simulink model "det3x3_HDL"  (R2024a)
settings: Solver=VariableStepAuto  StartTime=0.0  StopTime=100e-9  RelTol=1e-3
undefined symbols (not defined in the file or in its folder): S, vsva2197, xcvc1902
libraries: hdlBasic x32, hdlSSR x1, vmcUtilities x1
settings Model: Creator=catalinb  LastModifiedBy=sdegala
settings DebuggingCC: UnconnectedInputMsg=warning  UnconnectedOutputMsg=warning  UnconnectedLineMsg=warning
settings ModelReferenceCC: EnableRefExpFcnMdlSchedulingChecks=on
settings RTWCC: GPUComputeCapability=3.5  DLArmComputeVersion=19.05

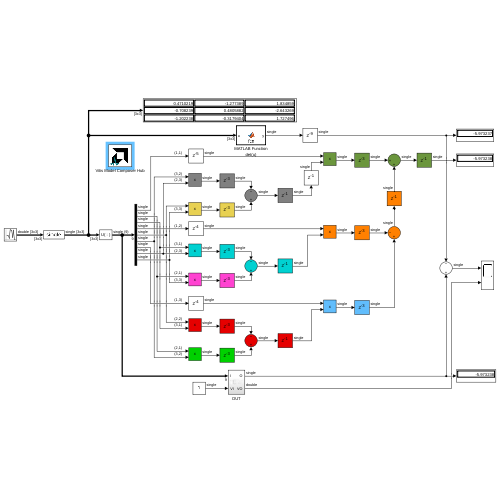
[thumbnail: Simulink's stored preview of the top-level diagram]
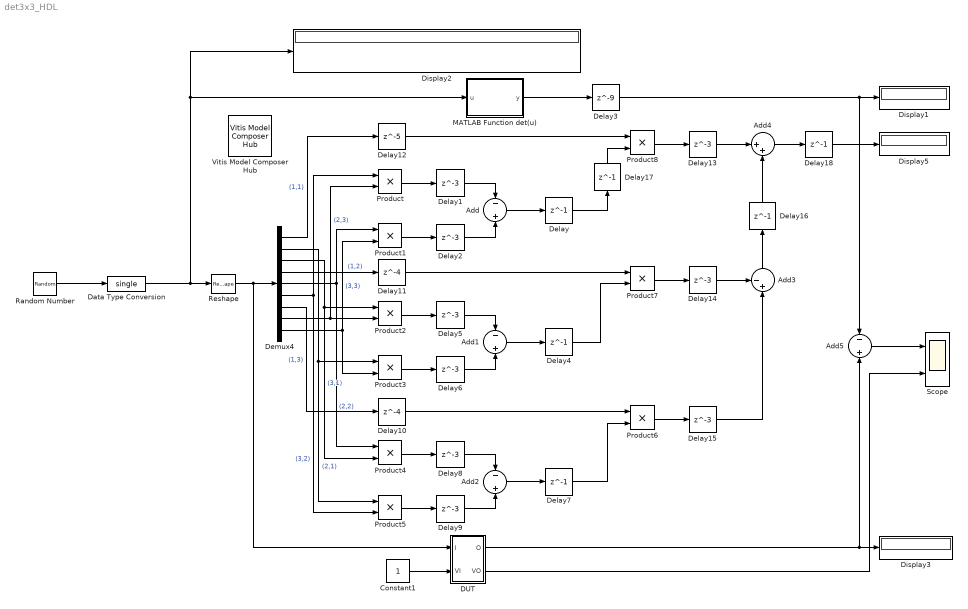
== system det3x3_HDL ==
  Add{,1..2,5} (4 alike) : Sum  Inputs=-|+
  Add3 : Sum  Inputs=-+|
  Add4 : Sum  Inputs=|++
  Constant1 : Constant  OutDataTypeStr=single  SampleTime=1/805e6
  DUT : Subsystem
  Data Type Conversion : DataTypeConversion  OutDataTypeStr=single  SaturateOnIntegerOverflow=off  RndMeth=Floor
  Delay{,4,7,16..18} (6 alike) : Delay  DelayLength=1
  Delay{1..2,5..6,8..9,13..15} (9 alike) : Delay  DelayLength=3
  Delay10 : Delay  DelayLength=4
  Delay11 : Delay  DelayLength=4
  Delay12 : Delay  DelayLength=5
  Delay3 : Delay  DelayLength=9
  Demux4 : Demux  Outputs=9
  Display{1..3,5} (4 alike) : Display
  MATLAB Function det(u) : MATLAB Function  TreatAsAtomicUnit=on
  Product{,1..8} (9 alike) : Product
  Random Number : RandomNumber  Mean=zeros(3,3)  Variance=ones(3,3)  Seed=reshape(1:9,3,3)  SampleTime=1.242e-9  VectorParams1D=off
  Reshape : Reshape
  Scope : Scope  NumInputPorts=2
  Vitis Model Composer Hub : vmcUtilities/Vitis Model Composer Hub  Tag=genX  CodeGeneration=off  SubsystemName=DUT  BlockHierPath=det3x3_HDL/DUT  CompilationType=HDLCompilation  SubsystemType=HDLNode  ExportTypeV2=IP Catalog  StartColumn=1  NumberOfColumns=1  TargetDirectory=./netlist  exportDesign=on  analyzeDesign=off  validateDesignOnHw=off  ExportType=HDL  IpVendor=xilinx.com  IpLibrary=hls  IpVersion=1.0  IpHWLanguage=Verilog  AieCompilerOptions={}  AieSimulatorOptions={}  CreateTestbench=on  TestbenchStackSize=10  RunRtlSim=off  RunCSim=off  RunAieSim=off  AieSimTimeout=50000  RunAieSimProfiling=off  LaunchVitisAnalyzer=off  PlotOutput=off  RunX86Sim=off  X86SimTimeout=10  GenHwImage=off  GenLibadfXo=on  GenHwValidationCode=off  PlatformType=Specify Platform  Platform=/proj/xbuilds/SWIP/9999.0_0905_1841/installs/lin64/2025.2/Vitis/base_platforms/xilinx_vck190_base_202520_1/xilinx_vck190_base_202520_1.xpfm  HwSystemType=Baremetal  HwValidationTarget=hw  ProjDevice=Versal VCK190 Evaluation Platform (xcvc1902-vsva2197-2MP-e-S)  ProjDevicePart=xcvc1902-vsva2197-2MP-e-S  AIEType=AIE  SamplePeriod=-1  ClockFrequency=200  DataPathParallelism=1  xilinxfamily=versalaicore  part=xcvc1902  speed=-2MP-e-S  package=vsva2197  directory=./netlist/ip/DUT/src  testbench=on  incr_netlist=off  synthesis_tool=Vivado  clock_wrapper=Clock Enables  dbl_ovrd=According to Block Masks  dcm_input_clock_period=10  sysclk_period=1.242  simulink_period=1.242e-9  eval_field=0  IPInfoJsonString="{\"DUTSubsystemName\":\"DUT\",\"HDLSubsystem\":{\"SubsystemName\":\"DUT\",\"IPName\":\"Subsystem\",\"IPLibrary\":\"VMC\",\"IPVendor\":\"User Company\",\"IPVersion\":\"1.0\",\"TargetDirectory\":\"./netlist\",\"SubsystemDir\":\"./netlist/ip/DUT\",\"FreqHz\":\"805152979.066\"},\"SubsystemTag\":\"HDLNode\"}"  LogFileName=/proj/xhdhdstaff5/sdegala/Head1/HEAD/ModelComposer_Sept16/Vitis_Model_Composer/Examples/HDL/Floating_Point/3x3_Matrix_Determinant/netlist/model_composer.log  NThreads=4  IPConfigFile=/tmp/vmctmp-9769773316677438567/det3x3_HDL_ipconfig.json
  wires:
  Add/1 -> Delay/1
  Product/1 -> Delay1/1
  Delay1/1 -> Add/1
  Product1/1 -> Delay2/1
  Delay2/1 -> Add/2
  Delay/1 -> Delay17/1
  MATLAB Function det(u)/1(y) -> Delay3/1
  Delay3/1 -> Add5/1, Display1/1
  Reshape/1 -> DUT/1(" I "), Demux4/1
  Demux4/1 -> Delay12/1  "(1,1)"
  Demux4/4 -> Delay11/1  "(1,2)"
  Demux4/7 -> Delay10/1  "(1,3)"
  Demux4/2 -> Product3/1, Product5/1  "(2,1)"
  Demux4/5 -> Product4/1, Product1/1  "(2,2)"
  Demux4/9 -> Product3/2, Product1/2  "(3,3)"
  Demux4/6 -> Product/1, Product5/2  "(3,2)"
  Demux4/8 -> Product/2, Product2/2  "(2,3)"
  Random Number/1 -> Data Type Conversion/1
  Delay4/1 -> Product7/2
  Delay6/1 -> Add1/2
  Product3/1 -> Delay6/1
  Delay5/1 -> Add1/1
  Product2/1 -> Delay5/1
  Add1/1 -> Delay4/1
  Demux4/3 -> Product4/2, Product2/1  "(3,1)"
  Add2/1 -> Delay7/1
  Product4/1 -> Delay8/1
  Delay8/1 -> Add2/1
  Product5/1 -> Delay9/1
  Delay9/1 -> Add2/2
  Delay7/1 -> Product6/2
  Delay10/1 -> Product6/1
  Delay11/1 -> Product7/1
  Delay12/1 -> Product8/1
  Product8/1 -> Delay13/1
  Product7/1 -> Delay14/1
  Product6/1 -> Delay15/1
  Delay14/1 -> Add3/1
  Delay15/1 -> Add3/2
  Add4/1 -> Delay18/1
  Delay16/1 -> Add4/2
  Add3/1 -> Delay16/1
  Delay13/1 -> Add4/1
  Delay18/1 -> Display5/1
  Delay17/1 -> Product8/2
  Constant1/1 -> DUT/2(" VI ")
  DUT/1(" O ") -> Add5/2, Display3/1
  Add5/1 -> Scope/1
  Data Type Conversion/1 -> MATLAB Function det(u)/1(u), Display2/1, Reshape/1
  DUT/2(" VO ") -> Scope/2

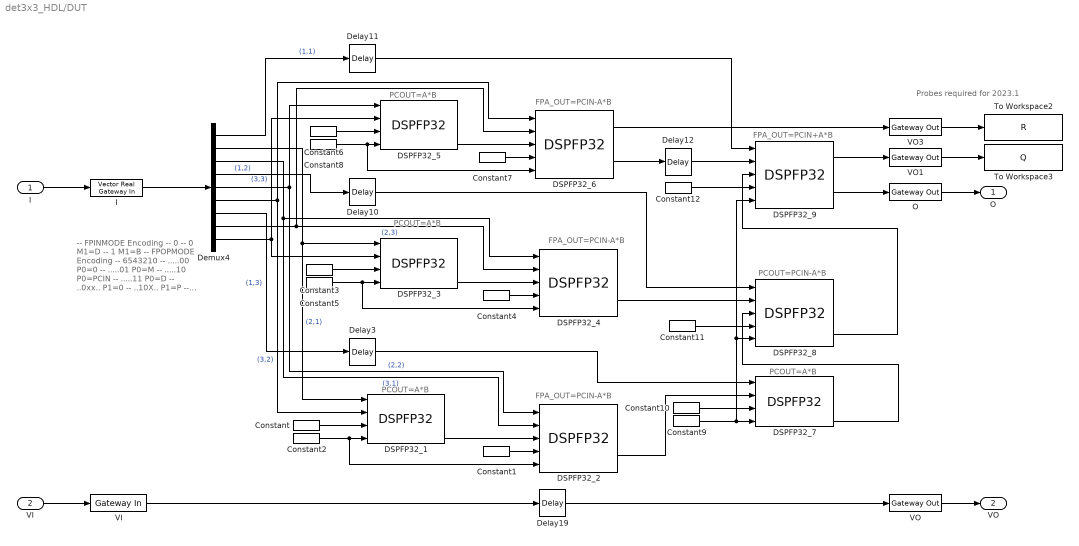
== system det3x3_HDL/DUT ==
  note: Probes required for 2023.1
  note: FPA_OUT=PCIN-A*B
  note: PCOUT=A*B
  note: -- FPINMODE Encoding
      | -- 0
      | -- 0 M1=D
      | -- 1 M1=B
      |
      | -- FPOPMODE Encoding
      | -- 6543210
      | -- .....00 P0=0
      | -- .....01 P0=M
      | -- .....10 P0=PCIN
      | -- .....11 P0=D
      |
      | -- ..0xx.. P1=0
      | -- ..10X.. P1=P
      | -- ..110.. P1=C
      | -- ..111.. P1=PCIN
      |
      | -- 00..... FPA_OUT=P0+P1
      | -- 01..... FPA_OUT=-P0+P1
      | -- 10..... FPA_OUT=P0-P1
      | -- 11..... FPA_OUT=-P0-P1
  note: PCOUT=A*B
  note: PCOUT=PCIN-A*B
  note: FPA_OUT=PCIN+A*B
  note: PCOUT=A*B
  note: PCOUT=A*B
  note: FPA_OUT=PCIN-A*B
  note: FPA_OUT=PCIN-A*B
  " I " : Inport
  " VI " : Inport  Port=2
  Constant{,3,6,10} (4 alike) : hdlBasic/Constant  const=1  gui_display_data_type=Fixed-point  arith_type=Unsigned  n_bits=7  bin_pt=0  preci_type=Single  exp_width=8  frac_width=24  explicit_period=off  period=1  XmcBlockStatus=1  maskContainerNames=tabcontainer1  block_type=constant  block_config=sysgen:Constant_config
  Constant{1,4,7,11} (4 alike) : hdlBasic/Constant  const=61  gui_display_data_type=Fixed-point  arith_type=Unsigned  n_bits=7  bin_pt=0  preci_type=Single  exp_width=8  frac_width=24  explicit_period=off  period=1  XmcBlockStatus=1  maskContainerNames=tabcontainer1  block_type=constant  block_config=sysgen:Constant_config
  Constant12 : hdlBasic/Constant  const=29  gui_display_data_type=Fixed-point  arith_type=Unsigned  n_bits=7  bin_pt=0  preci_type=Single  exp_width=8  frac_width=24  explicit_period=off  period=1  XmcBlockStatus=1  maskContainerNames=tabcontainer1  block_type=constant  block_config=sysgen:Constant_config
  Constant{2,5,8..9} (4 alike) : hdlBasic/Constant  const=1  gui_display_data_type=Fixed-point  arith_type=Unsigned  n_bits=1  bin_pt=0  preci_type=Single  exp_width=8  frac_width=24  explicit_period=off  period=1  XmcBlockStatus=1  maskContainerNames=tabcontainer1  block_type=constant  block_config=sysgen:Constant_config
  DSPFP32_{1,3,5,7} (4 alike) : hdlBasic/DSPFP32   use_a=Direct from a port  use_b=Direct from b port  a_fptype=B32  b_d_fptype=B32  xl_useadderonly=off  xl_dynamicmult=off  use_c=off  use_d=off  rst_all=off  en_all=off  use_pcin=off  use_fpainvalid=off  use_fpaoverflow=off  use_fpaunderflow=off  use_fpminvalid=off  use_fpmoverflow=off  use_fpmunderflow=off  use_acout=off  use_bcout=off  bcascsel=B  use_pcout=on  pcoutsel=FPM  pipeline_a=1  pipeline_acout=1  pipeline_fpcreg=3  pipeline_fpopmreg=1  pipeline_fpbreg=on  pipeline_fpa_preg=on  pipeline_fpm_preg=on  pipeline_fpdreg=on  pipeline_fpmpipereg=on  pipeline_fpinmodereg=on  rst_a=off  rst_b=off  rst_c=off  rst_fpmpipe=off  rst_fpm=off  rst_fpa=off  rst_d=off  rst_fpinmode=off  rst_fpopmode=off  en_a1=off  en_a2=off  en_b=off  en_c=off  en_fpmpipe=off  en_fpm=off  en_fpa=off  en_fpopmode=off  en_fpinmode=off  en_d=off  fpinmode_inverted=off  fpopmode_inverted=off  fpopmode_inverted_value='0000000'  is_rsta_inverted=off  is_rstb_inverted=off  is_rstc_inverted=off  is_rstd_inverted=off  is_rstfpa_inverted=off  is_rstfpinmode_inverted=off  is_rstfpmpipe_inverted=off  is_rstfpm_inverted=off  is_rstfpopmode_inverted=off  simulation_type=fast_sim  simulation_model=sysgen:dspfp32_macro  is_clk_inverted=false  reset_mode=SYNC  XmcBlockStatus=1  maskContainerNames=tabcontainer1  block_type=dspfp32  block_config=sysgen:DSPFP32_config  block_height=1080  block_width=800
  DSPFP32_2 : hdlBasic/DSPFP32   use_a=Direct from a port  use_b=Direct from b port  a_fptype=B32  b_d_fptype=B32  xl_useadderonly=off  xl_dynamicmult=off  use_c=off  use_d=off  rst_all=off  en_all=off  use_pcin=on  use_fpainvalid=off  use_fpaoverflow=off  use_fpaunderflow=off  use_fpminvalid=off  use_fpmoverflow=off  use_fpmunderflow=off  use_acout=off  use_bcout=off  bcascsel=B  use_pcout=off  pcoutsel=FPM  pipeline_a=1  pipeline_acout=1  pipeline_fpcreg=3  pipeline_fpopmreg=1  pipeline_fpbreg=on  pipeline_fpa_preg=on  pipeline_fpm_preg=on  pipeline_fpdreg=on  pipeline_fpmpipereg=on  pipeline_fpinmodereg=on  rst_a=off  rst_b=off  rst_c=off  rst_fpmpipe=off  rst_fpm=off  rst_fpa=off  rst_d=off  rst_fpinmode=off  rst_fpopmode=off  en_a1=off  en_a2=off  en_b=off  en_c=off  en_fpmpipe=off  en_fpm=off  en_fpa=off  en_fpopmode=off  en_fpinmode=off  en_d=off  fpinmode_inverted=off  fpopmode_inverted=off  fpopmode_inverted_value='0000000'  is_rsta_inverted=off  is_rstb_inverted=off  is_rstc_inverted=off  is_rstd_inverted=off  is_rstfpa_inverted=off  is_rstfpinmode_inverted=off  is_rstfpmpipe_inverted=off  is_rstfpm_inverted=off  is_rstfpopmode_inverted=off  simulation_type=fast_sim  simulation_model=sysgen:dspfp32_macro  is_clk_inverted=false  reset_mode=SYNC  XmcBlockStatus=1  maskContainerNames=tabcontainer1  block_type=dspfp32  block_config=sysgen:DSPFP32_config  block_height=1080  block_width=800
  DSPFP32_4 : hdlBasic/DSPFP32   use_a=Direct from a port  use_b=Direct from b port  a_fptype=B32  b_d_fptype=B32  xl_useadderonly=off  xl_dynamicmult=off  use_c=off  use_d=off  rst_all=off  en_all=off  use_pcin=on  use_fpainvalid=off  use_fpaoverflow=off  use_fpaunderflow=off  use_fpminvalid=off  use_fpmoverflow=off  use_fpmunderflow=off  use_acout=off  use_bcout=off  bcascsel=B  use_pcout=off  pcoutsel=FPM  pipeline_a=1  pipeline_acout=1  pipeline_fpcreg=3  pipeline_fpopmreg=1  pipeline_fpbreg=on  pipeline_fpa_preg=on  pipeline_fpm_preg=on  pipeline_fpdreg=on  pipeline_fpmpipereg=on  pipeline_fpinmodereg=on  rst_a=off  rst_b=off  rst_c=off  rst_fpmpipe=off  rst_fpm=off  rst_fpa=off  rst_d=off  rst_fpinmode=off  rst_fpopmode=off  en_a1=off  en_a2=off  en_b=off  en_c=off  en_fpmpipe=off  en_fpm=off  en_fpa=off  en_fpopmode=off  en_fpinmode=off  en_d=off  fpinmode_inverted=off  fpopmode_inverted=off  fpopmode_inverted_value='0000000'  is_rsta_inverted=off  is_rstb_inverted=off  is_rstc_inverted=off  is_rstd_inverted=off  is_rstfpa_inverted=off  is_rstfpinmode_inverted=off  is_rstfpmpipe_inverted=off  is_rstfpm_inverted=off  is_rstfpopmode_inverted=off  simulation_type=fast_sim  simulation_model=sysgen:dspfp32_macro  is_clk_inverted=false  reset_mode=SYNC  XmcBlockStatus=1  maskContainerNames=tabcontainer1  block_type=dspfp32  block_config=sysgen:DSPFP32_config  block_height=1080  block_width=800
  DSPFP32_6 : hdlBasic/DSPFP32   use_a=Direct from a port  use_b=Direct from b port  a_fptype=B32  b_d_fptype=B32  xl_useadderonly=off  xl_dynamicmult=off  use_c=off  use_d=off  rst_all=off  en_all=off  use_pcin=on  use_fpainvalid=off  use_fpaoverflow=off  use_fpaunderflow=off  use_fpminvalid=off  use_fpmoverflow=off  use_fpmunderflow=off  use_acout=off  use_bcout=off  bcascsel=B  use_pcout=off  pcoutsel=FPM  pipeline_a=1  pipeline_acout=1  pipeline_fpcreg=3  pipeline_fpopmreg=1  pipeline_fpbreg=on  pipeline_fpa_preg=on  pipeline_fpm_preg=on  pipeline_fpdreg=on  pipeline_fpmpipereg=on  pipeline_fpinmodereg=on  rst_a=off  rst_b=off  rst_c=off  rst_fpmpipe=off  rst_fpm=off  rst_fpa=off  rst_d=off  rst_fpinmode=off  rst_fpopmode=off  en_a1=off  en_a2=off  en_b=off  en_c=off  en_fpmpipe=off  en_fpm=off  en_fpa=off  en_fpopmode=off  en_fpinmode=off  en_d=off  fpinmode_inverted=off  fpopmode_inverted=off  fpopmode_inverted_value='0000000'  is_rsta_inverted=off  is_rstb_inverted=off  is_rstc_inverted=off  is_rstd_inverted=off  is_rstfpa_inverted=off  is_rstfpinmode_inverted=off  is_rstfpmpipe_inverted=off  is_rstfpm_inverted=off  is_rstfpopmode_inverted=off  simulation_type=hybrid  simulation_model=sysgen:dspfp32_macro  is_clk_inverted=false  reset_mode=SYNC  XmcBlockStatus=1  maskContainerNames=tabcontainer1  block_type=dspfp32  block_config=sysgen:DSPFP32_config  block_height=1080  block_width=800
  DSPFP32_8 : hdlBasic/DSPFP32   use_a=Direct from a port  use_b=Direct from b port  a_fptype=B32  b_d_fptype=B32  xl_useadderonly=off  xl_dynamicmult=off  use_c=off  use_d=off  rst_all=off  en_all=off  use_pcin=on  use_fpainvalid=off  use_fpaoverflow=off  use_fpaunderflow=off  use_fpminvalid=off  use_fpmoverflow=off  use_fpmunderflow=off  use_acout=off  use_bcout=off  bcascsel=B  use_pcout=on  pcoutsel=FPA  pipeline_a=1  pipeline_acout=1  pipeline_fpcreg=3  pipeline_fpopmreg=1  pipeline_fpbreg=on  pipeline_fpa_preg=on  pipeline_fpm_preg=on  pipeline_fpdreg=on  pipeline_fpmpipereg=on  pipeline_fpinmodereg=on  rst_a=off  rst_b=off  rst_c=off  rst_fpmpipe=off  rst_fpm=off  rst_fpa=off  rst_d=off  rst_fpinmode=off  rst_fpopmode=off  en_a1=off  en_a2=off  en_b=off  en_c=off  en_fpmpipe=off  en_fpm=off  en_fpa=off  en_fpopmode=off  en_fpinmode=off  en_d=off  fpinmode_inverted=off  fpopmode_inverted=off  fpopmode_inverted_value='0000000'  is_rsta_inverted=off  is_rstb_inverted=off  is_rstc_inverted=off  is_rstd_inverted=off  is_rstfpa_inverted=off  is_rstfpinmode_inverted=off  is_rstfpmpipe_inverted=off  is_rstfpm_inverted=off  is_rstfpopmode_inverted=off  simulation_type=fast_sim  simulation_model=sysgen:dspfp32_macro  is_clk_inverted=false  reset_mode=SYNC  XmcBlockStatus=1  maskContainerNames=tabcontainer1  block_type=dspfp32  block_config=sysgen:DSPFP32_config  block_height=1080  block_width=800
  DSPFP32_9 : hdlBasic/DSPFP32   use_a=Direct from a port  use_b=Direct from b port  a_fptype=B32  b_d_fptype=B32  xl_useadderonly=off  xl_dynamicmult=off  use_c=off  use_d=off  rst_all=off  en_all=off  use_pcin=on  use_fpainvalid=off  use_fpaoverflow=off  use_fpaunderflow=off  use_fpminvalid=off  use_fpmoverflow=off  use_fpmunderflow=off  use_acout=off  use_bcout=off  bcascsel=B  use_pcout=off  pcoutsel=FPM  pipeline_a=1  pipeline_acout=1  pipeline_fpcreg=3  pipeline_fpopmreg=1  pipeline_fpbreg=on  pipeline_fpa_preg=on  pipeline_fpm_preg=on  pipeline_fpdreg=on  pipeline_fpmpipereg=on  pipeline_fpinmodereg=on  rst_a=off  rst_b=off  rst_c=off  rst_fpmpipe=off  rst_fpm=off  rst_fpa=off  rst_d=off  rst_fpinmode=off  rst_fpopmode=off  en_a1=off  en_a2=off  en_b=off  en_c=off  en_fpmpipe=off  en_fpm=off  en_fpa=off  en_fpopmode=off  en_fpinmode=off  en_d=off  fpinmode_inverted=off  fpopmode_inverted=off  fpopmode_inverted_value='0000000'  is_rsta_inverted=off  is_rstb_inverted=off  is_rstc_inverted=off  is_rstd_inverted=off  is_rstfpa_inverted=off  is_rstfpinmode_inverted=off  is_rstfpmpipe_inverted=off  is_rstfpm_inverted=off  is_rstfpopmode_inverted=off  simulation_type=hybrid  simulation_model=sysgen:dspfp32_macro  is_clk_inverted=false  reset_mode=SYNC  XmcBlockStatus=1  maskContainerNames=tabcontainer1  block_type=dspfp32  block_config=sysgen:DSPFP32_config  block_height=1080  block_width=800
  Delay10 : hdlBasic/Delay  rst=off  en=off  latency=4  reg_retiming=off  XmcBlockStatus=1  maskContainerNames=group1  block_type=delay  block_config=sysgen:Delay_config
  Delay11 : hdlBasic/Delay  rst=off  en=off  latency=5  reg_retiming=off  XmcBlockStatus=1  maskContainerNames=group1  block_type=delay  block_config=sysgen:Delay_config
  Delay12 : hdlBasic/Delay  rst=off  en=off  latency=1  reg_retiming=off  XmcBlockStatus=1  maskContainerNames=group1  block_type=delay  block_config=sysgen:Delay_config
  Delay19 : hdlBasic/Delay  rst=off  en=off  latency=9  reg_retiming=off  XmcBlockStatus=1  maskContainerNames=group1  block_type=delay  block_config=sysgen:Delay_config
  Delay3 : hdlBasic/Delay  rst=off  en=off  latency=4  reg_retiming=off  XmcBlockStatus=1  maskContainerNames=group1  block_type=delay  block_config=sysgen:Delay_config
  Demux4 : Demux  Outputs=9
  I : hdlSSR/Vector Real Gateway In  gui_display_data_type=Floating-point  arith_type=Floating-point  n_bits=16  bin_pt=14  preci_type=Single  exp_width=8  frac_width=24  quantization="Round  (unbiased: +/- Inf)"  overflow=Saturate  period=1.242e-9  sg_ssr=9  UseAsADC=off  ADCChannel='1'  interface=None  automatic_assignment=on  address_offset=hex2dec('00')  intf_name=''  intf_description=''  default_value=0  timing_constraint=None  locs_specified=off  LOCs={}  io_standard={}  inherit_from_input=off  hdl_port=on  interface_prev=1  block_type=realgatewayin_ssr  XmcBlockStatus=1  sg_ssr_prev=9  maskContainerNames=group4  block_width_w=590  block_height_w=670  block_width=640  block_height=850
  O : hdlBasic/Gateway Out  inherit_from_input=on  bool_to_boolean=off  hdl_port=on  rows=1  columns=1  UseAsDAC=off  DACChannel='1'  interface=None  automatic_assignment=on  address_offset=hex2dec('00')  intf_name=''  intf_description=''  timing_constraint=None  locs_specified=off  LOCs={}  io_standard={}  XmcBlockStatus=1  maskContainerNames=group4  block_type=gatewayout  block_config=sysgen:gateway_out_config  block_width_w=590  block_height_w=620  block_width=620  block_height=750
  To Workspace2 : ToWorkspace  VariableName=R  SampleTime=-1
  To Workspace3 : ToWorkspace  VariableName=Q  SampleTime=-1
  VI : hdlBasic/Gateway In  gui_display_data_type=Boolean  arith_type=Boolean  n_bits=16  bin_pt=14  preci_type=Single  exp_width=8  frac_width=24  rows=1  columns=1  quantization="Round  (unbiased: +/- Inf)"  overflow=Saturate  period=1.242e-9  UseAsADC=off  ADCChannel='1'  interface=None  automatic_assignment=on  address_offset=hex2dec('00')  intf_name=''  intf_description=''  default_value=0  timing_constraint=None  locs_specified=off  LOCs={}  io_standard={}  inherit_from_input=off  hdl_port=on  XmcBlockStatus=1  maskContainerNames=group4  block_type=gatewayin  block_config=sysgen:gateway_in_config  block_width_w=590  block_height_w=620  block_width=640  block_height=850
  VO : hdlBasic/Gateway Out  inherit_from_input=off  bool_to_boolean=off  hdl_port=on  rows=1  columns=1  UseAsDAC=off  DACChannel='1'  interface=None  automatic_assignment=on  address_offset=hex2dec('00')  intf_name=''  intf_description=''  timing_constraint=None  locs_specified=off  LOCs={}  io_standard={}  XmcBlockStatus=1  maskContainerNames=group4  block_type=gatewayout  block_config=sysgen:gateway_out_config  block_width_w=590  block_height_w=620  block_width=620  block_height=750
  VO1 : hdlBasic/Gateway Out  inherit_from_input=off  bool_to_boolean=off  hdl_port=off  rows=1  columns=1  UseAsDAC=off  DACChannel='1'  interface=None  automatic_assignment=on  address_offset=hex2dec('00')  intf_name=''  intf_description=''  timing_constraint=None  locs_specified=off  LOCs={}  io_standard={}  XmcBlockStatus=1  maskContainerNames=group4  block_type=gatewayout  block_config=sysgen:gateway_out_config  block_width_w=590  block_height_w=620  block_width=620  block_height=750
  VO3 : hdlBasic/Gateway Out  inherit_from_input=off  bool_to_boolean=off  hdl_port=off  rows=1  columns=1  UseAsDAC=off  DACChannel='1'  interface=None  automatic_assignment=on  address_offset=hex2dec('00')  intf_name=''  intf_description=''  timing_constraint=None  locs_specified=off  LOCs={}  io_standard={}  XmcBlockStatus=1  maskContainerNames=group4  block_type=gatewayout  block_config=sysgen:gateway_out_config  block_width_w=590  block_height_w=620  block_width=620  block_height=750
  " O " : Outport
  " VO " : Outport  Port=2
  wires:
  VO/1 -> " VO "/1
  Delay19/1 -> VO/1
  VI/1 -> Delay19/1
  " I "/1 -> I/1
  I/1 -> Demux4/1
  " VI "/1 -> VI/1
  O/1 -> " O "/1
  Delay12/1 -> DSPFP32_9/2
  Delay11/1 -> DSPFP32_9/1
  Demux4/5 -> DSPFP32_5/1, DSPFP32_2/1  "(2,2)"
  Demux4/1 -> Delay11/1  "(1,1)"
  Demux4/9 -> DSPFP32_5/2, DSPFP32_3/2  "(3,3)"
  DSPFP32_4/2 -> DSPFP32_8/2
  Demux4/4 -> Delay10/1  "(1,2)"
  Delay10/1 -> DSPFP32_8/1
  DSPFP32_6/2 -> Delay12/1
  Demux4/3 -> DSPFP32_2/2, DSPFP32_4/1  "(3,1)"
  Demux4/8 -> DSPFP32_4/2, DSPFP32_6/2  "(2,3)"
  Delay3/1 -> DSPFP32_7/1
  Demux4/6 -> DSPFP32_6/1, DSPFP32_1/2  "(3,2)"
  Demux4/2 -> DSPFP32_1/1, DSPFP32_3/1  "(2,1)"
  Demux4/7 -> Delay3/1  "(1,3)"
  DSPFP32_1/3 -> DSPFP32_2/3
  DSPFP32_7/3 -> DSPFP32_8/3
  DSPFP32_8/3 -> DSPFP32_9/3
  DSPFP32_9/2 -> O/1
  Constant/1 -> DSPFP32_1/3
  Constant1/1 -> DSPFP32_2/4
  Constant2/1 -> DSPFP32_2/5, DSPFP32_1/4
  Constant5/1 -> DSPFP32_3/4, DSPFP32_4/5
  Constant4/1 -> DSPFP32_4/4
  Constant3/1 -> DSPFP32_3/3
  DSPFP32_3/3 -> DSPFP32_4/3
  Constant8/1 -> DSPFP32_6/5, DSPFP32_5/4
  Constant7/1 -> DSPFP32_6/4
  Constant6/1 -> DSPFP32_5/3
  DSPFP32_5/3 -> DSPFP32_6/3
  Constant9/1 -> DSPFP32_7/4, DSPFP32_8/5, DSPFP32_9/5
  Constant10/1 -> DSPFP32_7/3
  Constant11/1 -> DSPFP32_8/4
  Constant12/1 -> DSPFP32_9/4
  VO1/1 -> To Workspace3/1
  VO3/1 -> To Workspace2/1
  DSPFP32_2/2 -> DSPFP32_7/2
  DSPFP32_6/1 -> VO3/1
  DSPFP32_9/1 -> VO1/1

== matlab function det3x3_HDL/MATLAB Function det(u) ==
  data: u input; y output
function y = fcn(u)

y = det(u);
